simulink model "section_4_2"  (R2021b)
settings: Solver=VariableStepAuto  StartTime=0.0  StopTime=2000  RelTol=1e-3
values from neighbouring files (symbols this model uses):
  C1_z_den_quant = quant(C1_z_den, q)    [lab3.m]
  C1_z_num_quant = quant(C1_z_num, q)    [lab3.m]
  C2_z_den_quant = quant(C2_z_den, q)    [lab3.m]
  C2_z_num_quant = quant(C2_z_num, q)    [lab3.m]
  C3_z_den_quant = quant(C3_z_den, q)    [lab3.m]
  C3_z_num_quant = quant(C3_z_num, q)    [lab3.m]
  K_quant = quant(K, q)    [lab3.m]
  Pz_den = cell2mat(Pz.Denominator)    [lab3.m]
  Pz_num = cell2mat(Pz.Numerator)    [lab3.m]
  T = 0.1    [lab3.m]
settings Model: Creator=varunsampat  LastModifiedBy=varunsampat

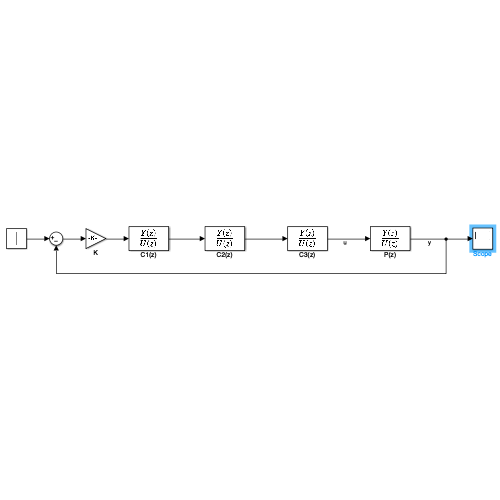
[thumbnail: Simulink's stored preview of the top-level diagram]
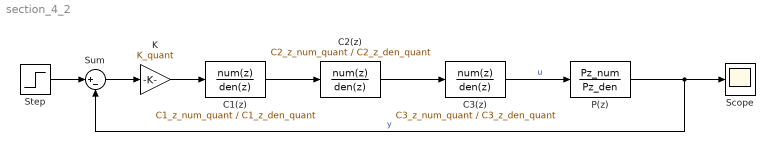
== system section_4_2 ==
  C1(z) : DiscreteTransferFcn  Numerator=C1_z_num_quant  Denominator=C1_z_den_quant  SampleTime=T
  C2(z) : DiscreteTransferFcn  Numerator=C2_z_num_quant  Denominator=C2_z_den_quant  SampleTime=T
  C3(z) : DiscreteTransferFcn  Numerator=C3_z_num_quant  Denominator=C3_z_den_quant  SampleTime=T
  K : Gain  Gain=K_quant
  P(z) : DiscreteTransferFcn  Numerator=Pz_num  Denominator=Pz_den
  Scope : Scope
  Step : Step  SampleTime=T
  Sum : Sum  Inputs=|+-
  wires:
  C3(z)/1 -> P(z)/1  "u"
  Sum/1 -> K/1
  P(z)/1 -> Sum/2, Scope/1  "y"
  Step/1 -> Sum/1
  K/1 -> C1(z)/1
  C1(z)/1 -> C2(z)/1
  C2(z)/1 -> C3(z)/1
